simulink model "simulation"  (R2020b)
settings: Solver=VariableStepAuto  StartTime=0.0  StopTime=20  RelTol=1e-3
undefined symbols (not defined in the file or in its folder): PQini, qini
libraries: pid_lib x1
settings Model: Creator=kt012  LastModifiedBy=kt012

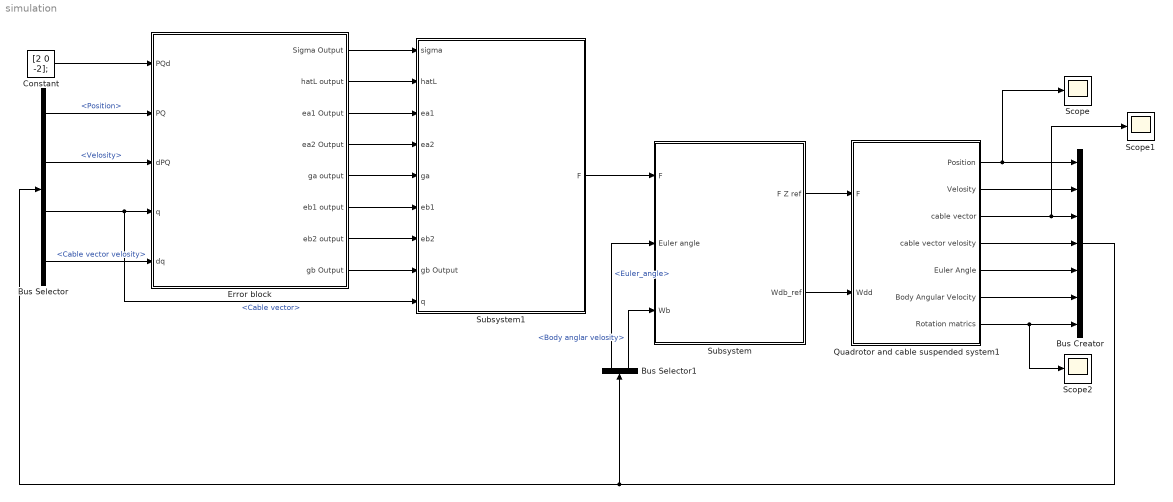
== system simulation ==
  Bus Creator : BusCreator  Inputs=7
  Bus Selector : BusSelector  OutputSignals=Position,Velosity,Cable vector,Cable vector velosity
  Bus Selector1 : BusSelector  OutputSignals=Euler_angle,Body anglar velosity
  Constant : Constant  Value=[2 0 -2];
  Error block : Subsystem
  Quadrotor and cable suspended system1 : Subsystem
  Scope : Scope
  Scope1 : Scope
  Scope2 : Scope
  Subsystem : Subsystem
  Subsystem1 : Subsystem
  wires:
  Error block/1(Sigma Output) -> Subsystem1/1(sigma)
  Error block/2(hatL output) -> Subsystem1/2(hatL)
  Error block/3(ea1 Output) -> Subsystem1/3(ea1)
  Error block/4(ea2 Output) -> Subsystem1/4(ea2)
  Error block/5(ga output) -> Subsystem1/5(ga)
  Error block/6(eb1 output) -> Subsystem1/6(eb1)
  Error block/7(eb2 output) -> Subsystem1/7(eb2)
  Subsystem1/1(F) -> Subsystem/1(F)
  Bus Creator/1 -> Bus Selector/1, Bus Selector1/1
  Bus Selector/1 -> Error block/2(PQ)  "<Position>"
  Bus Selector/2 -> Error block/3(dPQ)  "<Velosity>"
  Bus Selector/3 -> Subsystem1/9(q), Error block/4(q)  "<Cable vector>"
  Bus Selector/4 -> Error block/5(dq)  "<Cable vector velosity>"
  Constant/1 -> Error block/1(PQd)
  Error block/8(gb Output) -> Subsystem1/8(gb Output)
  Quadrotor and cable suspended system1/4(cable vector velosity) -> Bus Creator/4
  Quadrotor and cable suspended system1/3(cable vector) -> Scope1/1, Bus Creator/3
  Quadrotor and cable suspended system1/2(Velosity) -> Bus Creator/2
  Quadrotor and cable suspended system1/1(Position) -> Scope/1, Bus Creator/1
  Quadrotor and cable suspended system1/5(Euler Angle) -> Bus Creator/5
  Quadrotor and cable suspended system1/6(Body Angular Velocity) -> Bus Creator/6
  Quadrotor and cable suspended system1/7(Rotation matrics) -> Scope2/1, Bus Creator/7
  Subsystem/1(F Z ref) -> Quadrotor and cable suspended system1/1(F)
  Subsystem/2(Wdb_ref) -> Quadrotor and cable suspended system1/2(Wdd)
  Bus Selector1/2 -> Subsystem/3(Wb)  "<Body anglar velosity>"
  Bus Selector1/1 -> Subsystem/2(Euler angle)  "<Euler_angle>"

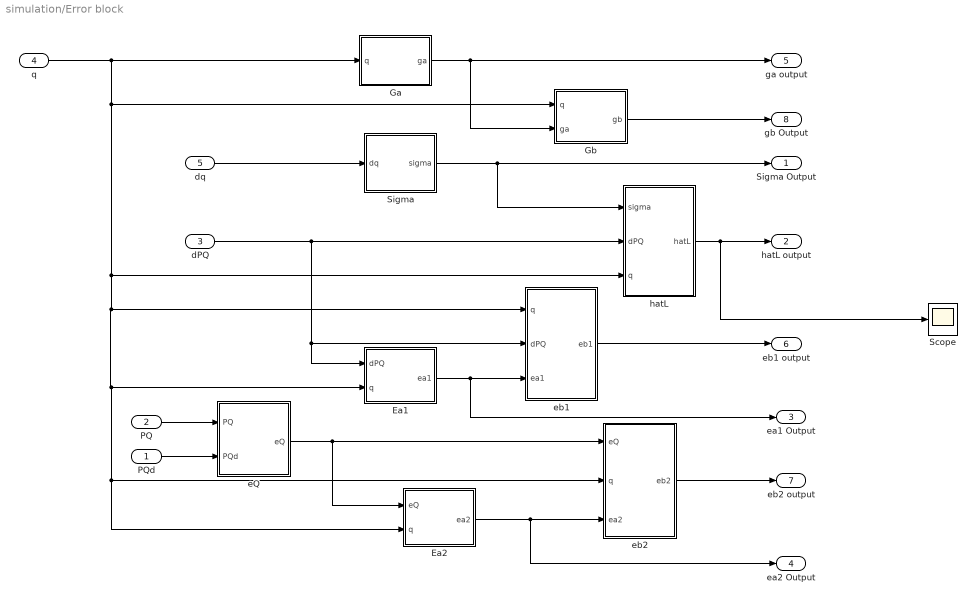
== system simulation/Error block ==
  PQd : Inport
  PQ : Inport  Port=2
  dPQ : Inport  Port=3
  q : Inport  Port=4
  dq : Inport  Port=5
  Ea1 : MATLAB Function  TreatAsAtomicUnit=on
  Ea2 : MATLAB Function  TreatAsAtomicUnit=on
  Ga : MATLAB Function  TreatAsAtomicUnit=on
  Gb : MATLAB Function  TreatAsAtomicUnit=on
  Scope : Scope
  Sigma : MATLAB Function  TreatAsAtomicUnit=on
  eQ : MATLAB Function  TreatAsAtomicUnit=on
  eb1 : MATLAB Function  TreatAsAtomicUnit=on
  eb2 : MATLAB Function  TreatAsAtomicUnit=on
  hatL : MATLAB Function  TreatAsAtomicUnit=on
  Sigma Output : Outport
  hatL output : Outport  Port=2
  ea1 Output : Outport  Port=3
  ea2 Output : Outport  Port=4
  ga output : Outport  Port=5
  eb1 output : Outport  Port=6
  eb2 output : Outport  Port=7
  gb Output : Outport  Port=8
  wires:
  hatL/1(hatL) -> Scope/1, hatL output/1
  dq/1 -> Sigma/1(dq)
  eb1/1(eb1) -> eb1 output/1
  Ea2/1(ea2) -> ea2 Output/1, eb2/3(ea2)
  PQ/1 -> eQ/1(PQ)
  Sigma/1(sigma) -> hatL/1(sigma), Sigma Output/1
  eQ/1(eQ) -> Ea2/1(eQ), eb2/1(eQ)
  Ea1/1(ea1) -> ea1 Output/1, eb1/3(ea1)
  q/1 -> Ga/1(q), Gb/1(q), hatL/3(q), eb1/1(q), Ea1/2(q), eb2/2(q), Ea2/2(q)
  PQd/1 -> eQ/2(PQd)
  eb2/1(eb2) -> eb2 output/1
  Ga/1(ga) -> Gb/2(ga), ga output/1
  dPQ/1 -> hatL/2(dPQ), eb1/2(dPQ), Ea1/1(dPQ)
  Gb/1(gb) -> gb Output/1

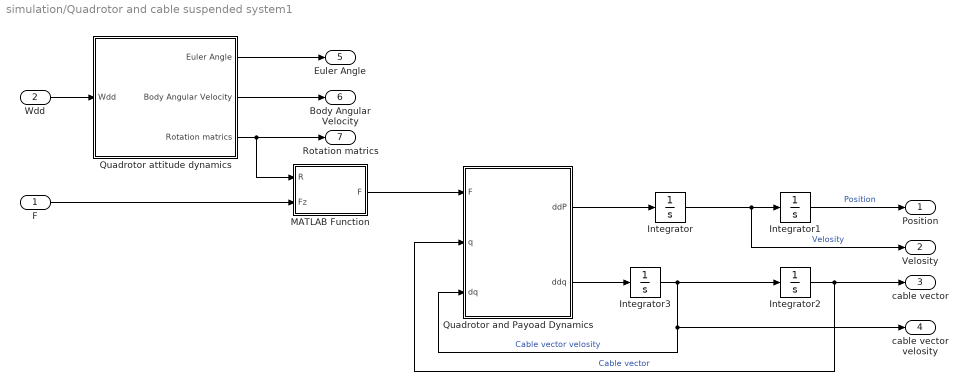
== system simulation/Quadrotor and cable suspended system1 ==
  F : Inport
  Wdd : Inport  Port=2
  Integrator : Integrator  InitialCondition=[0 0 0]
  Integrator1 : Integrator  InitialCondition=PQini
  Integrator2 : Integrator  InitialCondition=qini
  Integrator3 : Integrator  InitialCondition=[0 0 0]
  MATLAB Function : MATLAB Function  TreatAsAtomicUnit=on
  Quadrotor and Payoad Dynamics : Subsystem
  Quadrotor attitude dynamics : Subsystem
  Position : Outport
  Velosity : Outport  Port=2
  cable vector : Outport  Port=3
  cable vector velosity : Outport  Port=4
  Euler Angle : Outport  Port=5
  Body Angular Velocity : Outport  Port=6
  Rotation matrics : Outport  Port=7
  wires:
  F/1 -> MATLAB Function/2(Fz)
  Quadrotor and Payoad Dynamics/1(ddP) -> Integrator/1
  Integrator2/1 -> Quadrotor and Payoad Dynamics/2(q), cable vector/1  "Cable vector"
  Integrator/1 -> Integrator1/1, Velosity/1  "Velosity"
  Integrator1/1 -> Position/1  "Position"
  Quadrotor and Payoad Dynamics/2(ddq) -> Integrator3/1
  Integrator3/1 -> Quadrotor and Payoad Dynamics/3(dq), cable vector velosity/1, Integrator2/1  "Cable vector velosity"
  Wdd/1 -> Quadrotor attitude dynamics/1(Wdd)
  Quadrotor attitude dynamics/1(Euler Angle) -> Euler Angle/1
  Quadrotor attitude dynamics/2(Body Angular Velocity) -> Body Angular Velocity/1
  Quadrotor attitude dynamics/3(Rotation matrics) -> Rotation matrics/1, MATLAB Function/1(R)
  MATLAB Function/1(F) -> Quadrotor and Payoad Dynamics/1(F)

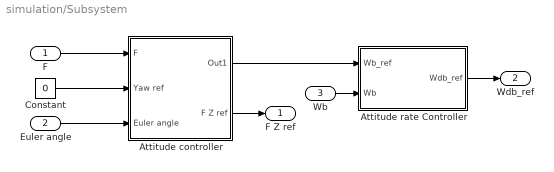
== system simulation/Subsystem ==
  F : Inport
  Euler angle : Inport  Port=2
  Wb : Inport  Port=3
  Attitude controller : Subsystem
  Attitude rate Controller : Subsystem
  Constant : Constant  Value=0
  F Z ref : Outport
  Wdb_ref : Outport  Port=2
  wires:
  Wb/1 -> Attitude rate Controller/2(Wb)
  Attitude rate Controller/1(Wdb_ref) -> Wdb_ref/1
  F/1 -> Attitude controller/1(F)
  Attitude controller/1(Out1) -> Attitude rate Controller/1(Wb_ref)
  Attitude controller/2(F Z ref) -> F Z ref/1
  Constant/1 -> Attitude controller/2(Yaw ref)
  Euler angle/1 -> Attitude controller/3(Euler angle)

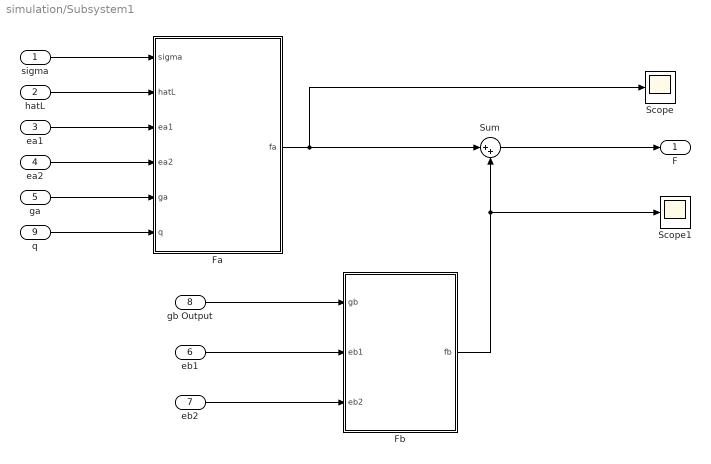
== system simulation/Subsystem1 ==
  sigma : Inport
  hatL : Inport  Port=2
  ea1 : Inport  Port=3
  ea2 : Inport  Port=4
  ga : Inport  Port=5
  eb1 : Inport  Port=6
  eb2 : Inport  Port=7
  gb Output : Inport  Port=8
  q : Inport  Port=9
  Fa : MATLAB Function  TreatAsAtomicUnit=on
  Fb : MATLAB Function  TreatAsAtomicUnit=on
  Scope : Scope
  Scope1 : Scope
  Sum : Sum  Inputs=|++
  F : Outport
  wires:
  eb1/1 -> Fb/2(eb1)
  Fa/1(fa) -> Scope/1, Sum/1
  Fb/1(fb) -> Sum/2, Scope1/1
  eb2/1 -> Fb/3(eb2)
  ga/1 -> Fa/5(ga)
  hatL/1 -> Fa/2(hatL)
  sigma/1 -> Fa/1(sigma)
  ea2/1 -> Fa/4(ea2)
  ea1/1 -> Fa/3(ea1)
  Sum/1 -> F/1
  gb Output/1 -> Fb/1(gb)
  q/1 -> Fa/6(q)

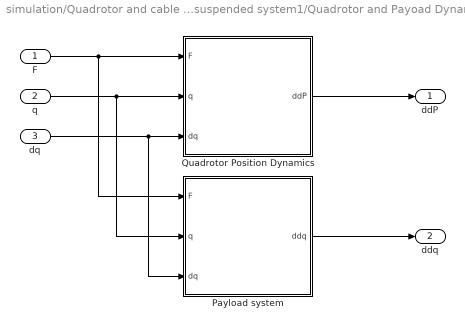
== system simulation/Quadrotor and cable suspended system1/Quadrotor and Payoad Dynamics ==
  F : Inport
  q : Inport  Port=2
  dq : Inport  Port=3
  Payload system : MATLAB Function  TreatAsAtomicUnit=on
  Quadrotor Position Dynamics : MATLAB Function  TreatAsAtomicUnit=on
  ddP : Outport
  ddq : Outport  Port=2
  wires:
  dq/1 -> Quadrotor Position Dynamics/3(dq), Payload system/3(dq)
  q/1 -> Quadrotor Position Dynamics/2(q), Payload system/2(q)
  F/1 -> Quadrotor Position Dynamics/1(F), Payload system/1(F)
  Quadrotor Position Dynamics/1(ddP) -> ddP/1
  Payload system/1(ddq) -> ddq/1

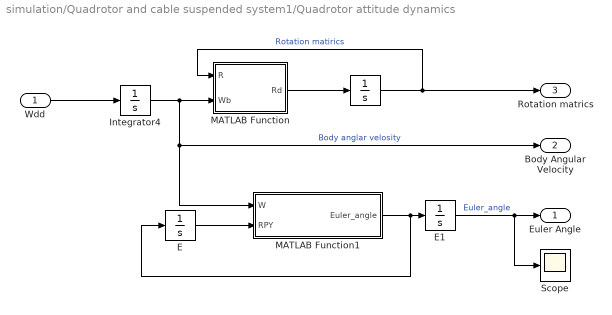
== system simulation/Quadrotor and cable suspended system1/Quadrotor attitude dynamics ==
  Wdd : Inport
  " " : Integrator  InitialCondition=[1 0 0; 0 1 0; 0 0 1];  ContinuousStateAttributes="\"\""
  E : Integrator  InitialCondition=[0 0 0];
  E1 : Integrator  InitialCondition=[0 0 0];
  Integrator4 : Integrator  InitialCondition=[0 0 0];  ContinuousStateAttributes='Body_anglar_velocity'
  MATLAB Function : MATLAB Function  TreatAsAtomicUnit=on
  MATLAB Function1 : MATLAB Function  TreatAsAtomicUnit=on
  Scope : Scope
  Euler Angle : Outport
  Body Angular Velocity : Outport  Port=2
  Rotation matrics : Outport  Port=3
  wires:
  Integrator4/1 -> Body Angular Velocity/1, MATLAB Function1/1(W), MATLAB Function/2(Wb)  "Body anglar velosity"
  MATLAB Function/1(Rd) -> " "/1
  E/1 -> MATLAB Function1/2(RPY)
  " "/1 -> Rotation matrics/1, MATLAB Function/1(R)  "Rotation matirics"
  MATLAB Function1/1(Euler_angle) -> E/1, E1/1
  E1/1 -> Scope/1, Euler Angle/1  "Euler_angle"
  Wdd/1 -> Integrator4/1

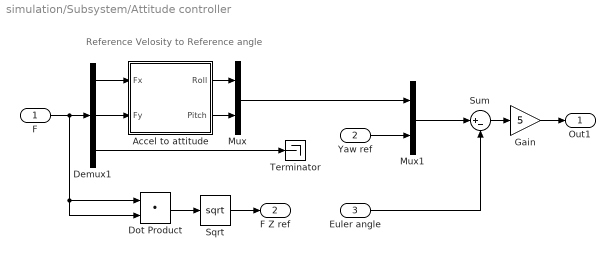
== system simulation/Subsystem/Attitude controller ==
  note: Reference Velosity to Reference angle
  F : Inport
  Yaw ref : Inport  Port=2
  Euler angle : Inport  Port=3
  Accel to attitude : MATLAB Function  TreatAsAtomicUnit=on
  Demux1 : Demux  Outputs=3
  Dot Product : DotProduct  InputSameDT=on  OutDataTypeStr=Inherit: Inherit via internal rule
  Gain : Gain  Gain=5
  Mux : Mux  Inputs=2
  Mux1 : Mux  Inputs=2
  Sqrt : Sqrt  SaturateOnIntegerOverflow=on
  Sum : Sum  Inputs=|+-
  Terminator : Terminator
  Out1 : Outport
  F Z ref : Outport  Port=2
  wires:
  Accel to attitude/2(Pitch) -> Mux/2
  Mux/1 -> Mux1/1
  Demux1/3 -> Terminator/1
  Demux1/1 -> Accel to attitude/1(Fx)
  F/1 -> Dot Product/1, Dot Product/2, Demux1/1
  Accel to attitude/1(Roll) -> Mux/1
  Demux1/2 -> Accel to attitude/2(Fy)
  Dot Product/1 -> Sqrt/1
  Sqrt/1 -> F Z ref/1
  Yaw ref/1 -> Mux1/2
  Mux1/1 -> Sum/1
  Euler angle/1 -> Sum/2
  Sum/1 -> Gain/1
  Gain/1 -> Out1/1

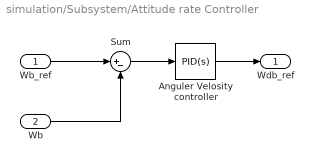
== system simulation/Subsystem/Attitude rate Controller ==
  Wb_ref : Inport
  Wb : Inport  Port=2
  Anguler Velosity controller : pid_lib/PID Controller  Controller=PID  Form=Parallel  TimeDomain=Continuous-time  UseExternalTs=off  SampleTime=-1  IntegratorMethod=Forward Euler  FilterMethod=Forward Euler  ControllerParametersSource=internal  P=1 * 180 / 3.14  I=0* 180 / 3.14  D=0 * 180 / 3.14  UseFilter=on  N=100  TunerSelectOption=Transfer Function Based (PID Tuner App)  InitialConditionSource=internal  InitialConditionForIntegrator=0  InitialConditionForFilter=0  DifferentiatorICPrevScaledInput=0  ExternalReset=none  TrackingMode=off  Kt=1  LimitOutput=off  SatLimitsSource=internal  UpperSaturationLimit=inf  LowerSaturationLimit=-inf  LinearizeAsGain=on  AntiWindupMode=none  Kb=1  POutMin=[]  POutMax=[]  IOutMin=[]  IOutMax=[]  DOutMin=[]  DOutMax=[]  NOutMin=[]  NOutMax=[]  SumOutMin=[]  SumOutMax=[]  SaturationOutMin=[]  SaturationOutMax=[]  PParamMin=[]  PParamMax=[]  IParamMin=[]  IParamMax=[]  DParamMin=[]  DParamMax=[]  NParamMin=[]  NParamMax=[]  KbParamMin=[]  KbParamMax=[]  KtParamMin=[]  KtParamMax=[]  KbOutMin=[]  KbOutMax=[]  KtOutMin=[]  KtOutMax=[]  IntegratorOutMin=[]  IntegratorOutMax=[]  FilterOutMin=[]  FilterOutMax=[]  SumI1OutMin=[]  SumI1OutMax=[]  SumI2OutMin=[]  SumI2OutMax=[]  SumI3OutMin=[]  SumI3OutMax=[]  SumI4OutMin=[]  SumI4OutMax=[]  SumDOutMin=[]  SumDOutMax=[]  DifferentiatorOutMin=[]  DifferentiatorOutMax=[]  FilterDiffOutCoefMin=[]  FilterDiffOutCoefMax=[]  ReciprocalOutMin=[]  ReciprocalOutMax=[]  SumDenOutMin=[]  SumDenOutMax=[]  SumNumOutMin=[]  SumNumOutMax=[]  DivideOutMin=[]  DivideOutMax=[]  UdiffTsProdOutMin=[]  UdiffTsProdOutMax=[]  NTsProdOutMin=[]  NTsProdOutMax=[]  UintegralTsProdOutMin=[]  UintegralTsProdOutMax=[]  UngainTsProdOutMin=[]  UngainTsProdOutMax=[]  IntegratorContinuousStateAttributes=''  IntegratorStateMustResolveToSignalObject=off  IntegratorRTWStateStorageClass=Auto  FilterContinuousStateAttributes=''  FilterStateMustResolveToSignalObject=off  FilterRTWStateStorageClass=Auto  ParallelPVariant=InternalParameters  IdealPVariant=Disabled  IVariant=InternalParameters  DVariant=InternalParameters  IntegratorVariant=Continuous  SatVariant=Disabled  AWVariant=Passthrough  PCopyVariant=Disabled  TRVariant=Disabled  FdbkBlocksVariant=Forward  IdealPFdbkVariant=Disabled  SatFdbkVariant=Disabled  DerivativeFilterVariant=ContFilter  NVariant=InternalParameters  NCopyVariant=Disabled  FilterICVariant=InternalICsFilter  IntegratorICVariant=InternalICs  ExternalResetVariant=Disabled  TRSumVariant=Passthrough  SumFdbkVariant=Disabled  SumVariant=Sum_PID  TsampFilterVariant=InternalTs  TsampNgainVariant=Passthrough  TsampIntegralVariant=Passthrough  ExternalSaturationOutDataTypeStr=Inherit: Same as second input
  Sum : Sum  Inputs=|+-
  Wdb_ref : Outport
  wires:
  Sum/1 -> Anguler Velosity controller/1
  Anguler Velosity controller/1 -> Wdb_ref/1
  Wb/1 -> Sum/2
  Wb_ref/1 -> Sum/1

== matlab function simulation/Error block/eb2 ==
  data: eQ input; q input; eb2 output; ea2 input
function eb2 = Eb2(eQ, q, ea2)
p = paramdef;
eb2 = p.kp*eQ - q*ea2;

== matlab function simulation/Error block/eQ ==
  data: PQ input; eQ output; PQd input
function eQ = fcn(PQ, PQd)

eQ = PQ - PQd;

== matlab function simulation/Error block/Gb ==
  data: gb output; q input; ga input
function gb = Gb(q, ga)
p = paramdef();
gb = p.G - q*ga;

== matlab function simulation/Quadrotor and cable suspended system1/Quadrotor and Payoad Dynamics/Payload system ==
  data: F input; ddq output; q input; dq input
function ddq = P_dynamics(F, q, dq)
p = paramdef;
Lddq = - q * ( p.L*In_pro(dq, dq) - In_pro(q, F)/p.mQ ) - F/p.mQ;

ddq = Lddq/p.L;

== matlab function simulation/Quadrotor and cable suspended system1/Quadrotor and Payoad Dynamics/Quadrotor Position Dynamics ==
  data: F input; ddP output; q input; dq input
function ddP = Q_dynamics(F, q, dq)
p = paramdef;
mQddP = p.mL/(p.mQ + p.mL) * q * ( p.mQ*p.L*In_pro(dq, dq) - In_pro(q, F) ) + p.mQ*p.G + F;

ddP = mQddP/p.mQ;

== matlab function simulation/Quadrotor and cable suspended system1/Quadrotor attitude dynamics/MATLAB Function1 ==
  data: W input; Euler_angle output; RPY input
function Euler_angle = fcn(W, RPY)
roll = RPY(1);
pitch = RPY(2);
yaw = RPY(3);
rollS = sin(roll); rollC = cos(roll);           
pitchS = sin(pitch); pitchC = cos(pitch);       


Euler_angle = pinv([1 0 -pitchS;
     0 rollC  pitchC * rollS;
     0 -rollS pitchC * rollC]) * W;

== matlab function simulation/Quadrotor and cable suspended system1/MATLAB Function ==
  data: R input; F output; Fz input
function F = fcn(R, Fz)
F = [R(1, 3) ; -R(2, 3); -R(3, 3)] * Fz;

== matlab function simulation/Subsystem/Attitude controller/Accel to attitude ==
  data: Fx input; Roll output; Pitch output; Fy input
function [Roll, Pitch]= fcn(Fx, Fy)
p = paramdef;
Roll = Fy/p.mQ * 3.14 / 180;
Pitch = Fx/p.mQ * 3.14 / 180;

== matlab function simulation/Quadrotor and cable suspended system1/Quadrotor attitude dynamics/MATLAB Function ==
  data: R input; Rd output; Wb input
function Rd = fcn(R, Wb)
wx = Wb(1);
wy = Wb(2);
wz = Wb(3);
Wb = [ 0    -wz   wy;
       wz    0   -wx;
      -wy    wx   0];
Rd = R * Wb;

== matlab function simulation/Subsystem1/Fa ==
  data: sigma input; hatL input; ea1 input; ea2 input; fa output; ga input; q input
function fa = Fa(sigma, hatL, ea1, ea2, ga, q)
p = paramdef;
fatmp = -(p.mL + p.mQ)/(p.kL*p.mL + p.kQ*p.mQ) * ...
     ( (p.kQ*p.mQ + p.kL*p.mL) * ga + sigma*hatL + ea2 + ea1);
fa = q * fatmp;

== matlab function simulation/Error block/Ga ==
  data: ga output; q input
function ga = Ga(q)
p = paramdef;
ga = In_pro(p.G, q);

== matlab function simulation/Error block/Ea1 ==
  data: dPQ input; ea1 output; q input
function ea1 = Ea1(dPQ, q)
p = paramdef;
ea1 = In_pro(p.kd*dPQ, q);

== matlab function simulation/Error block/Ea2 ==
  data: eQ input; q input; ea2 output
function ea2 = Ea2(eQ, q)
p = paramdef;
ea2 = In_pro(p.kp*eQ, q);

== matlab function simulation/Error block/Sigma ==
  data: dq input; sigma output
function sigma = Sig(dq)
p = paramdef;
sigma = (p.kQ - p.kL)*p.mQ*p.mL/(p.mQ + p.mL) * In_pro(dq, dq);

== matlab function simulation/Error block/hatL ==
  data: sigma input; dPQ input; hatL output; q input
function hatL = HATL(sigma, dPQ, q)
p = paramdef;
hatL = 1/p.SIGMA*Proj(sigma*In_pro(q, dPQ));

== matlab function simulation/Subsystem1/Fb ==
  data: gb input; eb1 input; eb2 input; fb output
function fb = Fb(gb, eb1, eb2)
p = paramdef;
fb = -1/p.kQ * ( eb2 + eb1 + (p.kQ*p.mQ + p.kL*p.mL) * gb);

== matlab function simulation/Error block/eb1 ==
  data: q input; dPQ input; eb1 output; ea1 input
function eb1 = Eb1(q, dPQ, ea1)
p = paramdef;
eb1 = p.kd*dPQ - q*ea1;
